simulink model "ClosedLoopStimUSB6009"  (R2016b)
settings: Solver=FixedStepDiscrete  StartTime=0.0  StopTime=inf  FixedStep=sCoreParams.core.stepPeriod  RelTol=1e-3  EnableMultiTasking=on
values from neighbouring files (symbols this model uses):
  sCoreParams = InitCoreParams_Dependent(sCoreParams)    [initializationScript.m]
undefined symbols (not defined in the file or in its folder): daq
libraries: slrtlib x5, dspswit3 x3, daqlib x2, xpcnilib x1
settings Model: DataTypeOverride=Double  MinMaxOverflowLogging=ForceOff  Creator=rzelmann  LastModifiedBy=rzelmann
settings SolverCC: EnableConcurrentExecution=on  ConcurrentTasks=on
settings DataIOCC: SaveFormat=StructureWithTime
settings OptimizationCC: DefaultParameterBehavior=Inlined  EfficientFloat2IntCast=on  LifeSpan=inf
settings DebuggingCC: UniqueDataStoreMsg=error  StrictBusMsg=ErrorOnBusTreatedAsVector  SFUnexpectedBacktrackingDiag=warning  SFNoUnconditionalDefaultTransitionDiag=warning  SFExecutionAtInitializationDiag=none
settings HardwareCC: ProdBitPerPointer=32  ProdBitPerSizeT=32  ProdBitPerPtrDiffT=32  ProdLargestAtomicFloat=None  ProdWordSize=32  ProdLongLongMode=on  ProdHWDeviceType=Generic->32-bit x86 compatible
settings ModelReferenceCC: ModelReferenceNumInstancesAllowed=Single
settings RTWCC: SystemTargetFile=slrt.tlc  TLCOptions="-axPCMaxOverloads=30            -axPCOverLoadLen=2 -axPCStartupFlag=5"  TemplateMakefile=slrt_default_tmf  Description=Simulink Real-Time  RTWCompilerOptimization=on
settings CodeAppCC: MaxIdLength=63
settings ConfigComp: CovMetricSettings=dw  CovHtmlReporting=on  CovSaveCumulativeToWorkspaceVar=on  CovSaveSingleToWorkspaceVar=on  CovExternalEMLEnable=off

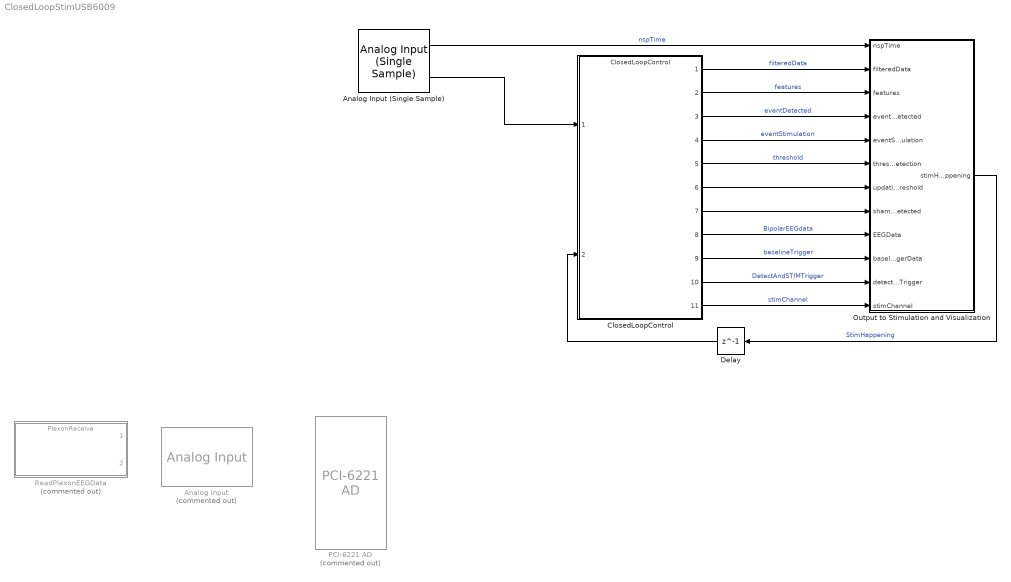
== system ClosedLoopStimUSB6009 ==
  Analog Input : daqlib/Analog Input  Commented=on  DeviceMenu=(none)  Device=ni Dev1 (USB-6009)  ObjConstructor=daq.createSession('ni')  NChannelsSelected=4  Channels=1$ai0$$Dev1$1$6$2$1$#1$ai1$$Dev1$1$6$2$1$#1$ai2$$Dev1$1$6$2$1$#1$ai3$$Dev1$1$6$2$1$#0$ai4$$Dev1$1$6$1$1$#0$ai5$$Dev1$1$6$1$1$#0$ai6$$Dev1$1$6$1$1$#0$ai7$$Dev1$1$6$1$1$#  NPorts=1 for all channels  SampleRate=2000  ActualRate=2000  ScansPerTrigger=100  OutputTimestamp=on  AcqMode=0  NumFrameBuffer=100  OutputTriggertime=off
  Analog Input (Single Sample) : daqlib/Analog Input (Single Sample)  DeviceMenu=(none)  Device=ni Dev1 (USB-6009)  ObjConstructor=daq.createSession('ni')  BlockSampleTime=.001  NChannelsSelected=8  Channels=1$ai0$$Dev1$1$6$1$1$#1$ai1$$Dev1$1$6$1$1$#1$ai2$$Dev1$1$6$1$1$#1$ai3$$Dev1$1$6$1$1$#1$ai4$$Dev1$1$7$1$1$#1$ai5$$Dev1$1$7$1$1$#1$ai6$$Dev1$1$7$1$1$#1$ai7$$Dev1$1$6$1$1$#  NPorts=1 for all channels  OutputTimestamp=on
  ClosedLoopControl : ModelReference  ModelNameDialog=ClosedLoopControl  SimulationMode=Normal  ModelReferenceVersion=1.628
  Delay : Delay  DelayLength=1  InitialCondition=0  InputProcessing=Columns as channels (frame based)  SampleTime=sCoreParams.core.stepPeriod
  Output to Stimulation and Visualization : Subsystem
  PCI-6221 AD : xpcnilib/A//D/M Series/PCI-6221 AD  Commented=on  channel=[1:16]  range=[5]  coupling=[0]  scantime=5e-6  sampletime=sCoreParams.core.stepPeriod  slot=-1
  ReadPlexonEEGData : ModelReference  Commented=on  ModelNameDialog=PlexonReceive.slx  SimulationMode=Normal  ModelReferenceVersion=1.11
  wires:
  Output to Stimulation and Visualization/1(stimHappening) -> Delay/1  "StimHappening"
  ClosedLoopControl/1 -> Output to Stimulation and Visualization/2(filteredData)  "filteredData"
  Analog Input (Single Sample)/1 -> Output to Stimulation and Visualization/1(nspTime)  "nspTime"
  ClosedLoopControl/4 -> Output to Stimulation and Visualization/5(eventStimulation)  "eventStimulation"
  ClosedLoopControl/6 -> Output to Stimulation and Visualization/7(updatingThreshold)
  ClosedLoopControl/8 -> Output to Stimulation and Visualization/9(EEGData)  "BipolarEEGdata"
  ClosedLoopControl/9 -> Output to Stimulation and Visualization/10(baselineTriggerData)  "baselineTrigger"
  ClosedLoopControl/10 -> Output to Stimulation and Visualization/11(detectStimTrigger)  "DetectAndSTIMTrigger"
  Delay/1 -> ClosedLoopControl/2
  ClosedLoopControl/11 -> Output to Stimulation and Visualization/12(stimChannel)  "stimChannel"
  ClosedLoopControl/7 -> Output to Stimulation and Visualization/8(shamDetected)
  ClosedLoopControl/5 -> Output to Stimulation and Visualization/6(thresholdUsedInDetection)  "threshold"
  ClosedLoopControl/3 -> Output to Stimulation and Visualization/4(eventDetected)  "eventDetected"
  ClosedLoopControl/2 -> Output to Stimulation and Visualization/3(features)  "features"
  Analog Input (Single Sample)/2 -> ClosedLoopControl/1

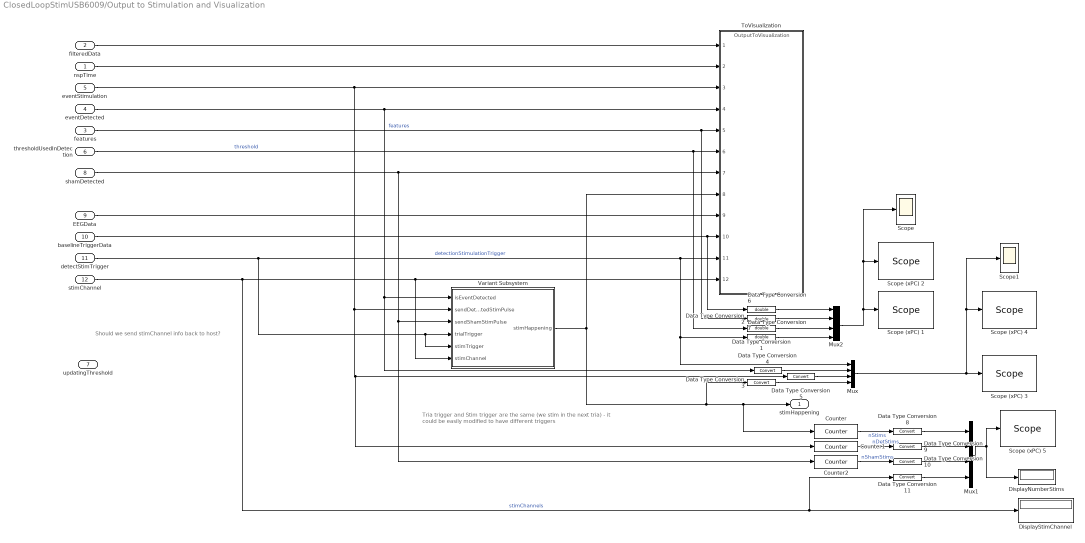
== system ClosedLoopStimUSB6009/Output to Stimulation and Visualization ==
  note: Should we send stimChannel info back to host?
  note: Tria trigger and Stim trigger are the same (we stim in the next tria)
      | - it could be easily modified to have different triggers
  nspTime : Inport
  filteredData : Inport  Port=2
  features : Inport  Port=3
  eventDetected : Inport  Port=4
  eventStimulation : Inport  Port=5
  thresholdUsedInDetection : Inport  Port=6
  updatingThreshold : Inport  Port=7
  shamDetected : Inport  Port=8
  EEGData : Inport  Port=9
  baselineTriggerData : Inport  Port=10  OutDataTypeStr=int32
  detectStimTrigger : Inport  Port=11  OutDataTypeStr=int32
  stimChannel : Inport  Port=12
  Counter : dspswit3/Counter  Direction=Up  CountEvent=Rising edge  CounterSize=User defined  MaxCount=1024  InitialCount=0  Output=Count  HitValue=32  ResetInput=off  SamplesPerFrame=1  Ts=1  CntDtype=int32  HitDtype=Logical
  Counter1 : dspswit3/Counter  Direction=Up  CountEvent=Rising edge  CounterSize=User defined  MaxCount=1024  InitialCount=0  Output=Count  HitValue=32  ResetInput=off  SamplesPerFrame=1  Ts=1  CntDtype=int32  HitDtype=Logical
  Counter2 : dspswit3/Counter  Direction=Up  CountEvent=Rising edge  CounterSize=User defined  MaxCount=1024  InitialCount=0  Output=Count  HitValue=32  ResetInput=off  SamplesPerFrame=1  Ts=1  CntDtype=int32  HitDtype=Logical
  Data Type Conversion{1..2,6..7} (4 alike) : DataTypeConversion  OutDataTypeStr=double
  Data Type Conversion{3..5,8..11} (7 alike) : DataTypeConversion
  DisplayNumberStims : Display
  DisplayStimChannel : Display
  Mux : Mux
  Mux1 : Mux
  Mux2 : Mux
  Scope : Scope
  Scope (xPC) 1 : slrtlib/Displays and Logging/Scope   scopeno=1  scopetype=Target  autostart=on  viewmode=Graphical sliding  formatstr='%15.6f'  grid=on  ylimits=[0,0]  nosamples=1000  noprepostsamples=0  interleave=1  triggermode=FreeRun  triggersignal=1  trigsignalfromport=on  triggerlevel=0.0  triggerslope=Rising  triggerscope=1  triggersample=0  filename=data.dat  mode=Lazy  writesize=512  autorestart=off  dynamicfilemode=off  maxwritefilesize=512*1024^2
  Scope (xPC) 2 : slrtlib/Displays and Logging/Scope   scopeno=2  scopetype=File  autostart=on  viewmode=Graphical redraw  formatstr='%15.6f'  grid=on  ylimits=[0,0]  nosamples=1000  noprepostsamples=-10  interleave=1  triggermode=FreeRun  triggersignal=1  trigsignalfromport=on  triggerlevel=0.0  triggerslope=Rising  triggerscope=1  triggersample=0  filename=featTh.dat  mode=Lazy  writesize=512  autorestart=off  dynamicfilemode=off  maxwritefilesize=512*1024^2
  Scope (xPC) 3 : slrtlib/Displays and Logging/Scope   scopeno=3  scopetype=Target  autostart=on  viewmode=Graphical sliding  formatstr='%15.6f'  grid=on  ylimits=[0,0]  nosamples=1000  noprepostsamples=0  interleave=1  triggermode=FreeRun  triggersignal=1  trigsignalfromport=on  triggerlevel=0.0  triggerslope=Rising  triggerscope=1  triggersample=0  filename=data.dat  mode=Lazy  writesize=512  autorestart=off  dynamicfilemode=off  maxwritefilesize=512*1024^2
  Scope (xPC) 4 : slrtlib/Displays and Logging/Scope   scopeno=4  scopetype=File  autostart=on  viewmode=Graphical redraw  formatstr='%15.6f'  grid=on  ylimits=[0,0]  nosamples=1000  noprepostsamples=-10  interleave=1  triggermode=FreeRun  triggersignal=1  trigsignalfromport=on  triggerlevel=0.0  triggerslope=Rising  triggerscope=1  triggersample=0  filename=detStim.dat  mode=Lazy  writesize=512  autorestart=off  dynamicfilemode=off  maxwritefilesize=512*1024^2
  Scope (xPC) 5 : slrtlib/Displays and Logging/Scope   scopeno=5  scopetype=Target  autostart=on  viewmode=Numerical  formatstr='%d'  grid=on  ylimits=[0,0]  nosamples=1000  noprepostsamples=0  interleave=1  triggermode=FreeRun  triggersignal=1  trigsignalfromport=on  triggerlevel=0.0  triggerslope=Rising  triggerscope=1  triggersample=0  filename=data.dat  mode=Lazy  writesize=512  autorestart=off  dynamicfilemode=off  maxwritefilesize=512*1024^2
  Scope1 : Scope
  ToVisualization : ModelReference  ModelNameDialog=OutputToVisualization  SimulationMode=Normal  ModelReferenceVersion=1.235
  Variant Subsystem : Subsystem  Variant=on
  stimHappening : Outport  OutDataTypeStr=boolean  SampleTime=sCoreParams.core.stepPeriod
  wires:
  eventDetected/1 -> Data Type Conversion4/1, Variant Subsystem/1(isEventDetected), ToVisualization/4
  nspTime/1 -> ToVisualization/2
  shamDetected/1 -> Counter2/1, Variant Subsystem/3(sendShamStimPulse), ToVisualization/7
  Variant Subsystem/1(stimHappening) -> ToVisualization/8, Data Type Conversion3/1, Counter/1, stimHappening/1
  eventStimulation/1 -> ToVisualization/3, Variant Subsystem/2(sendDetectedStimPulse), Counter1/1, Data Type Conversion5/1
  filteredData/1 -> ToVisualization/1
  EEGData/1 -> ToVisualization/9
  features/1 -> Data Type Conversion2/1, ToVisualization/5  "features"
  thresholdUsedInDetection/1 -> Data Type Conversion1/1, ToVisualization/6  "threshold"
  Data Type Conversion3/1 -> Mux/4
  Data Type Conversion4/1 -> Mux/2
  Mux2/1 -> Scope/1, Scope (xPC) 2/1, Scope (xPC) 1/1
  Mux/1 -> Scope1/1, Scope (xPC) 4/1, Scope (xPC) 3/1
  Data Type Conversion5/1 -> Mux/3
  baselineTriggerData/1 -> Data Type Conversion6/1, ToVisualization/10
  Data Type Conversion1/1 -> Mux2/3
  Data Type Conversion2/1 -> Mux2/2
  Data Type Conversion6/1 -> Mux2/1
  detectStimTrigger/1 -> Variant Subsystem/5(stimTrigger), Variant Subsystem/4(trialTrigger), Mux/1, Data Type Conversion7/1, ToVisualization/11  "detectionStimulationTrigger"
  Data Type Conversion7/1 -> Mux2/4
  stimChannel/1 -> Variant Subsystem/6(stimChannel), ToVisualization/12, Data Type Conversion11/1, DisplayStimChannel/1  "stimChannels"
  Counter/1 -> Data Type Conversion8/1  "nStims"
  Mux1/1 -> Scope (xPC) 5/1, DisplayNumberStims/1
  Counter1/1 -> Data Type Conversion9/1  "nDetStims"
  Counter2/1 -> Data Type Conversion10/1  "nShamStims"
  Data Type Conversion8/1 -> Mux1/1
  Data Type Conversion9/1 -> Mux1/2
  Data Type Conversion10/1 -> Mux1/3
  Data Type Conversion11/1 -> Mux1/4

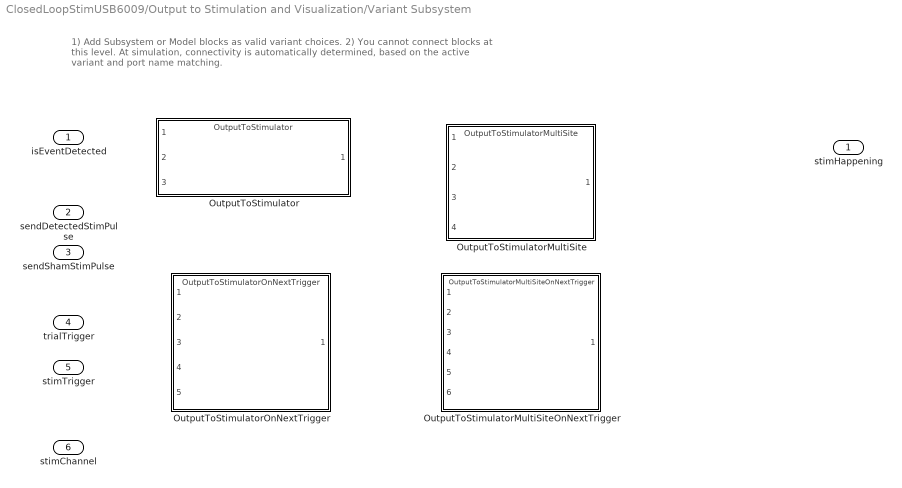
== system ClosedLoopStimUSB6009/Output to Stimulation and Visualization/Variant Subsystem ==
  note: 1) Add Subsystem or Model blocks as valid variant choices.
      | 2) You cannot connect blocks at this level. At simulation, connectivity is automatically
      | determined, based on the active variant and port name matching.
  isEventDetected : Inport
  sendDetectedStimPulse : Inport  Port=2
  sendShamStimPulse : Inport  Port=3
  trialTrigger : Inport  Port=4
  stimTrigger : Inport  Port=5
  stimChannel : Inport  Port=6  OutDataTypeStr=int32
  OutputToStimulator : ModelReference  ModelNameDialog=OutputToStimulator  SimulationMode=Normal  VariantControl=variantParams_STIMULATION_REALTIME  ModelReferenceVersion=1.30
  OutputToStimulatorMultiSite : ModelReference  ModelNameDialog=OutputToStimulatorMultiSite.slx  SimulationMode=Normal  VariantControl=variantParams_STIMULATION_MULTISITE_REALTIME  ModelReferenceVersion=1.45
  OutputToStimulatorMultiSiteOnNextTrigger : ModelReference  ModelNameDialog=OutputToStimulatorMultiSiteOnNextTrigger.slx  SimulationMode=Normal  VariantControl=variantParams_STIMULATION_MULTISITE_NEXTTRIGGER  ModelReferenceVersion=1.63
  OutputToStimulatorOnNextTrigger : ModelReference  ModelNameDialog=OutputToStimulatorOnNextTrigger  SimulationMode=Normal  VariantControl=variantParams_STIMULATION_ONNEXTTRIGGER  ModelReferenceVersion=1.45
  stimHappening : Outport
